simulink model "Lab3Simulink_Number1"  (R2023b)
settings: Solver=VariableStepAuto  StartTime=0.0  StopTime=20  RelTol=1e-3
values from neighbouring files (symbols this model uses):
  G1_den = [1 0 0]    [Lab3_Number1Codes.m]    (also in Problem2Group10.m)
  G1_num = [0 0 1]    [Lab3_Number1Codes.m]    (also in Problem2Group10.m = [1])
  G2_den = [1 1]    [Lab3_Number1Codes.m]    (also in Problem2Group10.m)
  G2_num = [0 1]    [Lab3_Number1Codes.m]    (also in Problem2Group10.m = [1])
  G3_den = [1 0]    [Lab3_Number1Codes.m]    (also in Problem2Group10.m)
  G3_num = [0 1]    [Lab3_Number1Codes.m]    (also in Problem2Group10.m = [1])
  H1_den = [1 0]    [Lab3_Number1Codes.m]    (also in Problem2Group10.m)
  H1_num = [0 1]    [Lab3_Number1Codes.m]    (also in Problem2Group10.m = [1])
  H2_den = [1 -1]    [Lab3_Number1Codes.m]    (also in Problem2Group10.m)
  H2_num = [0 1]    [Lab3_Number1Codes.m]    (also in Problem2Group10.m = [1])
  H3_den = [1 -2]    [Lab3_Number1Codes.m]    (also in Problem2Group10.m)
  H3_num = [0 1]    [Lab3_Number1Codes.m]    (also in Problem2Group10.m = [1])
  TF_den = conv(TF5_den,TF4_den)    [Lab3_Number1Codes.m]
  TF_num = conv(TF5_num, TF4_num)    [Lab3_Number1Codes.m]
settings Model: Creator=Asus  LastModifiedBy=Asus

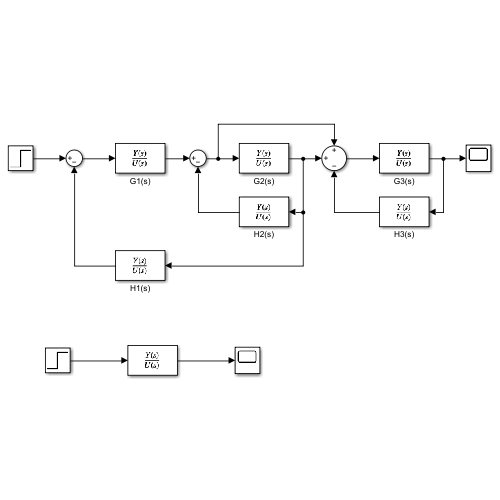
[thumbnail: Simulink's stored preview of the top-level diagram]
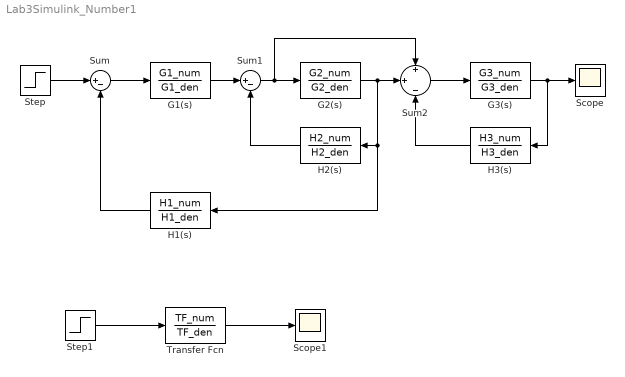
== system Lab3Simulink_Number1 ==
  G1(s) : TransferFcn  Numerator=G1_num  Denominator=G1_den
  G2(s) : TransferFcn  Numerator=G2_num  Denominator=G2_den
  G3(s) : TransferFcn  Numerator=G3_num  Denominator=G3_den
  H1(s) : TransferFcn  Numerator=H1_num  Denominator=H1_den
  H2(s) : TransferFcn  Numerator=H2_num  Denominator=H2_den
  H3(s) : TransferFcn  Numerator=H3_num  Denominator=H3_den
  Scope : Scope
  Scope1 : Scope
  Step : Step  Time=0  SampleTime=0
  Step1 : Step  Time=0  SampleTime=0
  Sum : Sum  Inputs=|+-
  Sum1 : Sum  Inputs=|+-
  Sum2 : Sum  Inputs=+|+|-
  Transfer Fcn : TransferFcn  Numerator=TF_num  Denominator=TF_den
  wires:
  Sum1/1 -> Sum2/1, G2(s)/1
  Step/1 -> Sum/1
  Sum/1 -> G1(s)/1
  G1(s)/1 -> Sum1/1
  G2(s)/1 -> H1(s)/1, H2(s)/1, Sum2/2
  Sum2/1 -> G3(s)/1
  G3(s)/1 -> H3(s)/1, Scope/1
  H3(s)/1 -> Sum2/3
  H2(s)/1 -> Sum1/2
  H1(s)/1 -> Sum/2
  Step1/1 -> Transfer Fcn/1
  Transfer Fcn/1 -> Scope1/1
